simulink model "SimpleMotorPositionController"  (R2019b)
settings: Solver=VariableStepAuto  StartTime=0.0  StopTime=10.0  RelTol=1e-3
undefined symbols (not defined in the file or in its folder): denc_mi, numc_mi
settings Model: Creator=Duin home  LastModifiedBy=Duin home

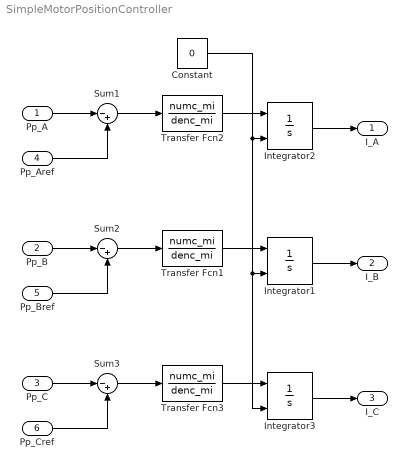
== system SimpleMotorPositionController ==
  Pp_A : Inport
  Pp_B : Inport  Port=2
  Pp_C : Inport  Port=3
  Pp_Aref : Inport  Port=4
  Pp_Bref : Inport  Port=5
  Pp_Cref : Inport  Port=6
  Constant : Constant  Value=0
  Integrator1 : Integrator  ExternalReset=rising  LimitOutput=on  UpperSaturationLimit=3  LowerSaturationLimit=-3
  Integrator2 : Integrator  ExternalReset=rising  LimitOutput=on  UpperSaturationLimit=3  LowerSaturationLimit=-3
  Integrator3 : Integrator  ExternalReset=rising  LimitOutput=on  UpperSaturationLimit=3  LowerSaturationLimit=-3
  Sum1 : Sum  Inputs=|-+  SaturateOnIntegerOverflow=on
  Sum2 : Sum  Inputs=|-+  SaturateOnIntegerOverflow=on
  Sum3 : Sum  Inputs=|-+  SaturateOnIntegerOverflow=on
  Transfer Fcn1 : TransferFcn  Numerator=numc_mi  Denominator=denc_mi
  Transfer Fcn2 : TransferFcn  Numerator=numc_mi  Denominator=denc_mi
  Transfer Fcn3 : TransferFcn  Numerator=numc_mi  Denominator=denc_mi
  I_A : Outport
  I_B : Outport  Port=2
  I_C : Outport  Port=3
  wires:
  Transfer Fcn2/1 -> Integrator2/1
  Constant/1 -> Integrator3/2, Integrator1/2, Integrator2/2
  Sum1/1 -> Transfer Fcn2/1
  Transfer Fcn1/1 -> Integrator1/1
  Transfer Fcn3/1 -> Integrator3/1
  Pp_A/1 -> Sum1/1
  Sum2/1 -> Transfer Fcn1/1
  Pp_B/1 -> Sum2/1
  Pp_C/1 -> Sum3/1
  Sum3/1 -> Transfer Fcn3/1
  Pp_Aref/1 -> Sum1/2
  Pp_Bref/1 -> Sum2/2
  Pp_Cref/1 -> Sum3/2
  Integrator2/1 -> I_A/1
  Integrator1/1 -> I_B/1
  Integrator3/1 -> I_C/1
